simulink model "st2"  (R2018b)
settings: Solver=ode45  StartTime=0.0  StopTime=20  RelTol=1e-3
settings Model: Creator=12732  LastModifiedBy=12732
settings DataIOCC: SaveFormat=Array

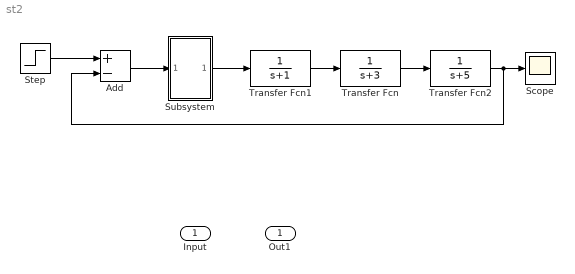
== system st2 ==
  Input : Inport
  Add : Sum  Inputs=+-
  Scope : Scope
  Step : Step  Before=1  SampleTime=0
  Subsystem : Subsystem  mask{Kp=5, Ti=0.658, Td=0.164}
  Transfer Fcn : TransferFcn  Denominator=[1 3]
  Transfer Fcn1 : TransferFcn  Denominator=[1 1]
  Transfer Fcn2 : TransferFcn  Denominator=[1 5]
  Out1 : Outport
  wires:
  Transfer Fcn/1 -> Transfer Fcn2/1
  Transfer Fcn1/1 -> Transfer Fcn/1
  Subsystem/1(Out1) -> Transfer Fcn1/1
  Transfer Fcn2/1 -> Add/2, Scope/1
  Step/1 -> Add/1
  Add/1 -> Subsystem/1(Input)

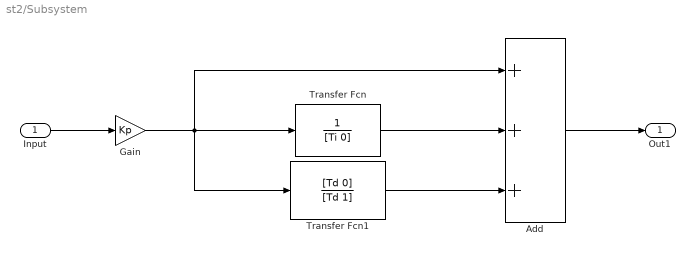
== system st2/Subsystem ==
  Input : Inport
  Add : Sum  Inputs=+++
  Gain : Gain  Gain=Kp
  Transfer Fcn : TransferFcn  Denominator=[Ti 0]
  Transfer Fcn1 : TransferFcn  Numerator=[Td 0]  Denominator=[Td 1]
  Out1 : Outport
  wires:
  Transfer Fcn1/1 -> Add/3
  Add/1 -> Out1/1
  Gain/1 -> Transfer Fcn1/1, Transfer Fcn/1, Add/1
  Transfer Fcn/1 -> Add/2
  Input/1 -> Gain/1
